simulink model "Problem1_dynamic_vibration_absorber"  (R2020b)
settings: Solver=VariableStepAuto  StartTime=0.0  StopTime=10  MaxStep=0.01  RelTol=1e-3
values from neighbouring files (symbols this model uses):
  b = 50    [Data.mat]
  K1 = 50    [Data.mat]
  K12 = 800    [Data.mat]
  M1 = 100    [Data.mat]
  M2 = 250    [Data.mat]
settings Model: Creator=vigne  LastModifiedBy=vigne
settings DataIOCC: ExternalInput=[t,Fin]  LoadExternalInput=on  SaveFormat=Array

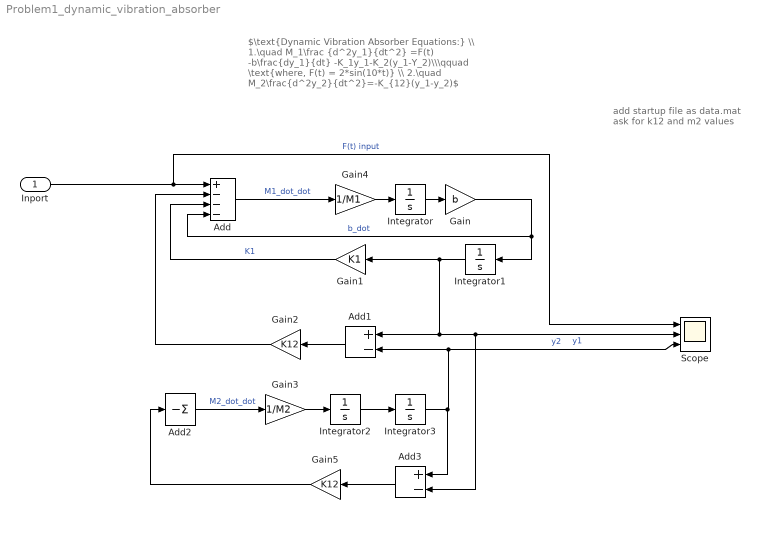
== system Problem1_dynamic_vibration_absorber ==
  note: add startup file as data.mat
      |
      | ask for k12 and m2 values
  note: $\text{Dynamic Vibration Absorber Equations:} \\ 1.\quad M_1\frac {d^2y_1}{dt^2} =F(t) -b\frac{dy_1}{dt} -K_1y_1-K_2(y_1-Y_2)\\\qquad \text{where, F(t) = 2*sin(10*t)} \\ 2.\quad M_2\frac{d^2y_2}{dt^2}=-K_{12}(y_1-y_2)$
  Inport : Inport
  Add : Sum  Inputs=+---
  Add1 : Sum  Inputs=+-
  Add2 : Sum  Inputs=-
  Add3 : Sum  Inputs=+-
  Gain : Gain  Gain=b
  Gain1 : Gain  Gain=K1
  Gain2 : Gain  Gain=K12
  Gain3 : Gain  Gain=1/M2
  Gain4 : Gain  Gain=1/M1
  Gain5 : Gain  Gain=K12
  Integrator{,1..3} (4 alike) : Integrator
  Scope : Scope  NumInputPorts=3
  wires:
  Add/1 -> Gain4/1  "M1_dot_dot"
  Integrator/1 -> Gain/1
  Integrator1/1 -> Add3/2, Scope/2, Add1/1, Gain1/1  "y1"
  Gain1/1 -> Add/3  "K1"
  Add1/1 -> Gain2/1
  Gain/1 -> Add/4, Integrator1/1  "b_dot"
  Add2/1 -> Gain3/1  "M2_dot_dot"
  Integrator2/1 -> Integrator3/1
  Gain4/1 -> Integrator/1
  Gain3/1 -> Integrator2/1
  Integrator3/1 -> Add3/1, Scope/3, Add1/2  "y2"
  Gain2/1 -> Add/2
  Add3/1 -> Gain5/1
  Gain5/1 -> Add2/1
  Inport/1 -> Scope/1, Add/1  "F(t) input"
